simulink model "FinalProjectSimulinkModel_OBSTACLE"  (R2023b)
settings: Solver=VariableStepAuto  StartTime=0.0  StopTime=17  RelTol=1e-3
values from neighbouring files (symbols this model uses):
  dq_d_COM = [0.75; 0; 0; 0; 0; 0]    [FinalProject_init.m]
  dq_d_COM_Jump = [10; 0; 20; 0; -30; 0]    [FinalProject_init.m]
  dq_d_COM_Jump_2 = [12; 0; 21.2; 0; -35.6; 0]    [FinalProject_init.m]
  dtMPC = 0.03    [FinalProject_init.m]
  firstStairDist = 0.26    [FinalProject_init.m]
  flight_gait_2 = [tcrouch2;fFofft2;rFofft2;rlandt2;flandt2; tImpact]    [FinalProject_init.m]
  flight_gait_t = [tcrouch;fFofft;rFofft;rlandt;flandt; tImpact]    [FinalProject_init.m]
  kd_swing = 10    [FinalProject_init.m]
  kp_swing = 300    [FinalProject_init.m]
  kStep = 0.001    [FinalProject_init.m]
  NMPC = 10    [FinalProject_init.m]
  offsets = [0;tSwing;tSwing;0]    [FinalProject_init.m]
  q_d_crouch = [q_hip_roll_f ... (first row only)    [FinalProject_init.m]
  q_d_impact = [q_hip_roll_i_f ... (first row only)    [FinalProject_init.m]
  q_d_stand = [q_hip_roll_i;q_hip_pitch_i;q_knee_i]    [FinalProject_init.m]
  q_hip_roll_i = 0    [FinalProject_init.m]
  Qmpc = diag([100 100 50 1000 1000 500 4 4 4 1 1 1 0])    [FinalProject_init.m]
  rFofft = 0.12+tcrouch    (= 1.12)    [FinalProject_init.m]
  rFofft2 = 0.12+tcrouch2    (= 1.42)    [FinalProject_init.m]
  Rmpc = 0.00001*eye(12)    [FinalProject_init.m]
  task = 6    [FinalProject_init.m]
  tcrouch = 1.0    (= 1)    [FinalProject_init.m]
  tcrouch2 = 1.3    [FinalProject_init.m]
  tCycle = 0.3    [FinalProject_init.m]
  tRamp = 0.5    [FinalProject_init.m]
  tRamp_Jump = 0.05    [FinalProject_init.m]
  tRamp_Jump2 = 0.08    [FinalProject_init.m]
  tSlow = 0.3    [FinalProject_init.m]
  tSwing = tCycle/2    (= 0.15)    [FinalProject_init.m]
  x0_Trunk = [0;0;z_trunk_i-.15; 0;-0.271;0]    [FinalProject_init.m]
undefined symbols (not defined in the file or in its folder): kStepTheta, X, Y, Z
libraries: sm_lib x199, nesl_utility x53
(part 1 of 6)
settings Model: Creator=Scott  LastModifiedBy=Scott

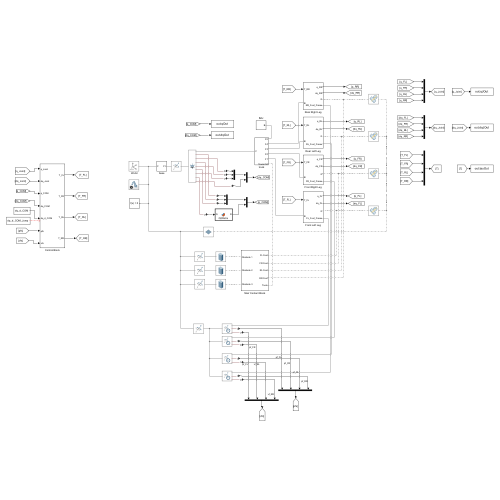
[thumbnail: Simulink's stored preview of the top-level diagram]
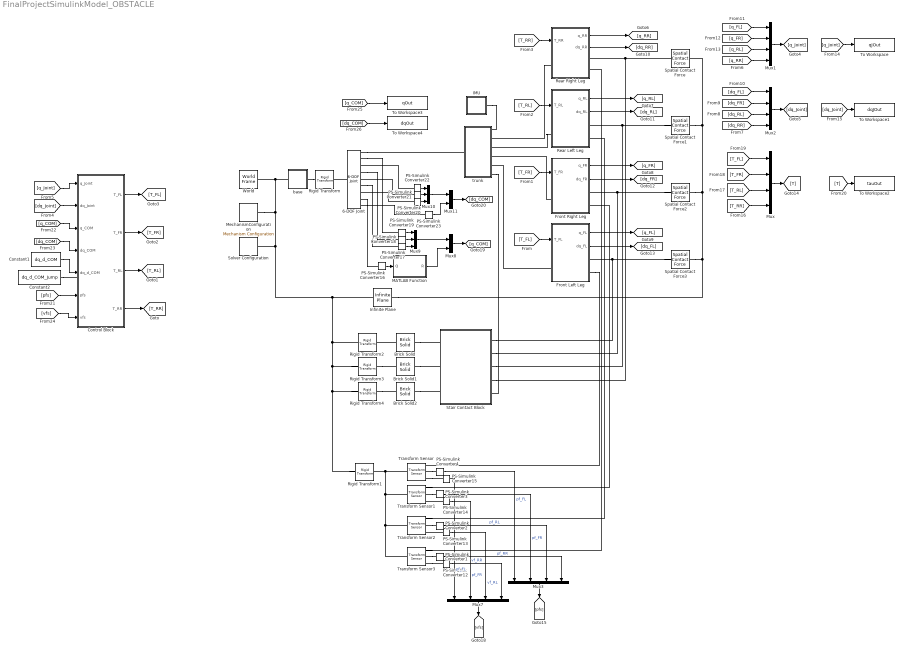
== system FinalProjectSimulinkModel_OBSTACLE ==
  6-DOF Joint : sm_lib/Joints/6-DOF Joint  JointMode=Normal  SenseConstraintForce=off  SenseConstraintForceX=off  SenseConstraintForceY=off  SenseConstraintForceZ=off  SenseConstraintTorque=off  SenseConstraintTorqueX=off  SenseConstraintTorqueY=off  SenseConstraintTorqueZ=off  SenseTotalForce=off  SenseTotalForceX=off  SenseTotalForceY=off  SenseTotalForceZ=off  SenseTotalTorque=off  SenseTotalTorqueX=off  SenseTotalTorqueY=off  SenseTotalTorqueZ=off  CompositeWrenchDir=FollowerOnBase  CompositeWrenchFrame=BaseFrame  PxEquilibriumPosition=0  PxEquilibriumPositionUnits=m  PxSpringStiffness=0  PxSpringStiffnessUnits=N/m  PxDampingCoefficient=0  PxDampingCoefficientUnits=N/(m/s)  PxTorqueActuationMode=NoTorque  PxMotionActuationMode=ComputedMotion  PxSensePosition=on  PxSenseVelocity=on  PxSenseAcceleration=off  PxSenseTorqueForce=off  PxSenseLowerLimitTorqueForce=off  PxSenseUpperLimitTorqueForce=off  PxLowerLimitSpecify=off  PxLowerLimitBound=-1  PxLowerLimitBoundUnits=m  PxLowerLimitStiffness=1e6  PxLowerLimitStiffnessUnits=N/m  PxLowerLimitDamping=1e3  PxLowerLimitDampingUnits=N/(m/s)  PxLowerLimitTransitionRegionWidth=1e-4  PxLowerLimitTransitionRegionWidthUnits=m  PxUpperLimitSpecify=off  PxUpperLimitBound=1  PxUpperLimitBoundUnits=m  PxUpperLimitStiffness=1e6  PxUpperLimitStiffnessUnits=N/m  PxUpperLimitDamping=1e3  PxUpperLimitDampingUnits=N/(m/s)  PxUpperLimitTransitionRegionWidth=1e-4  PxUpperLimitTransitionRegionWidthUnits=m  PxPositionTargetSpecify=off  PxPositionTargetPriority=High  PxPositionTargetValue=0  PxPositionTargetValueUnits=m  PxVelocityTargetSpecify=off  PxVelocityTargetPriority=High  PxVelocityTargetValue=0  PxVelocityTargetValueUnits=m/s  PyEquilibriumPosition=0  PyEquilibriumPositionUnits=m  PySpringStiffness=0  PySpringStiffnessUnits=N/m  PyDampingCoefficient=0  PyDampingCoefficientUnits=N/(m/s)  PyTorqueActuationMode=NoTorque  PyMotionActuationMode=ComputedMotion  PySensePosition=on  PySenseVelocity=on  PySenseAcceleration=off  PySenseTorqueForce=off  PySenseLowerLimitTorqueForce=off  PySenseUpperLimitTorqueForce=off  PyLowerLimitSpecify=off  PyLowerLimitBound=-1  PyLowerLimitBoundUnits=m  PyLowerLimitStiffness=1e6  PyLowerLimitStiffnessUnits=N/m  PyLowerLimitDamping=1e3  PyLowerLimitDampingUnits=N/(m/s)  PyLowerLimitTransitionRegionWidth=1e-4  PyLowerLimitTransitionRegionWidthUnits=m  PyUpperLimitSpecify=off  PyUpperLimitBound=1  PyUpperLimitBoundUnits=m  PyUpperLimitStiffness=1e6  PyUpperLimitStiffnessUnits=N/m  PyUpperLimitDamping=1e3  PyUpperLimitDampingUnits=N/(m/s)  PyUpperLimitTransitionRegionWidth=1e-4  PyUpperLimitTransitionRegionWidthUnits=m  PyPositionTargetSpecify=off  PyPositionTargetPriority=High  PyPositionTargetValue=0  PyPositionTargetValueUnits=m  PyVelocityTargetSpecify=off  PyVelocityTargetPriority=High  PyVelocityTargetValue=0  PyVelocityTargetValueUnits=m/s  PzEquilibriumPosition=0  PzEquilibriumPositionUnits=m  PzSpringStiffness=0  PzSpringStiffnessUnits=N/m  PzDampingCoefficient=0  PzDampingCoefficientUnits=N/(m/s)  PzTorqueActuationMode=NoTorque  PzMotionActuationMode=ComputedMotion  PzSensePosition=on  PzSenseVelocity=on  PzSenseAcceleration=off  PzSenseTorqueForce=off  PzSenseLowerLimitTorqueForce=off  PzSenseUpperLimitTorqueForce=off  PzLowerLimitSpecify=off  PzLowerLimitBound=-1  PzLowerLimitBoundUnits=m  PzLowerLimitStiffness=1e6  PzLowerLimitStiffnessUnits=N/m  PzLowerLimitDamping=1e3  PzLowerLimitDampingUnits=N/(m/s)  PzLowerLimitTransitionRegionWidth=1e-4  PzLowerLimitTransitionRegionWidthUnits=m  PzUpperLimitSpecify=off  PzUpperLimitBound=1  PzUpperLimitBoundUnits=m  PzUpperLimitStiffness=1e6  PzUpperLimitStiffnessUnits=N/m  PzUpperLimitDamping=1e3  PzUpperLimitDampingUnits=N/(m/s)  PzUpperLimitTransitionRegionWidth=1e-4  PzUpperLimitTransitionRegionWidthUnits=m  PzPositionTargetSpecify=on  PzPositionTargetPriority=High  PzPositionTargetValue=z_trunk_i  PzPositionTargetValueUnits=m  PzVelocityTargetSpecify=off  PzVelocityTargetPriority=High  PzVelocityTargetValue=0  PzVelocityTargetValueUnits=m/s  SphEqPosRotationMethod=None  SphEqPosRotationAngleUnits=deg  SphEqPosRotationStandardAxis=+Z  SphEqPosRotationAngle=0.0  SphEqPosRotationArbitraryAxis=[0 0 1]  SphEqPosFollAlignAxisA=+X  SphEqPosBaseAlignAxisA=+Y  SphEqPosFollAlignAxisB=+Y  SphEqPosBaseAlignAxisB=+Z  SphEqPosRotationSequenceAxes=FollowerAxes  SphEqPosRotationSequence=XYX  SphEqPosRotationSequenceAngles=[0 0 0]  SphEqPosRotationSequenceAnglesUnits=deg  SphEqPosRotationMatrix=[1 0 0; 0 1 0; 0 0 1]  SphEqPosQuaternion=[1 0 0 0]  SphSpringStiffness=0  SphSpringStiffnessUnits=N*m/deg  SphDampingCoefficient=0  SphDampingCoefficientUnits=N*m/(deg/s)  SphActuateTorqueX=off  SphActuateTorqueY=off  SphActuateTorqueZ=off  SphActuateTorque=off  SphTorqueActuationMode=NoTorque  SphMotionActuationMode=ComputedMotion  SphActuationFrame=BaseFrame  SphSensePosition=on  SphSenseVelocityX=off  SphSenseVelocityY=off  SphSenseVelocityZ=off  SphSenseVelocity=on  SphSenseAccelerationX=off  SphSenseAccelerationY=off  SphSenseAccelerationZ=off  SphSenseAcceleration=off  SphSenseTorqueX=off  SphSenseTorqueY=off  SphSenseTorqueZ=off  SphSenseTorqueForce=off  SphSenseLowerLimitTorqueMag=off  SphSenseUpperLimitTorqueMag=off  SphSensingFrame=BaseFrame  SphLowerLimitSpecify=off  SphLowerLimitBound=15  SphLowerLimitBoundUnits=deg  SphLowerLimitStiffness=1e4  SphLowerLimitStiffnessUnits=N*m/deg  SphLowerLimitDamping=10  SphLowerLimitDampingUnits=N*m/(deg/s)  SphLowerLimitTransitionRegionWidth=0.1  SphLowerLimitTransitionRegionWidthUnits=deg  SphUpperLimitSpecify=off  SphUpperLimitBound=45  SphUpperLimitBoundUnits=deg  SphUpperLimitStiffness=1e4  SphUpperLimitStiffnessUnits=N*m/deg  SphUpperLimitDamping=10  SphUpperLimitDampingUnits=N*m/(deg/s)  SphUpperLimitTransitionRegionWidth=0.1  SphUpperLimitTransitionRegionWidthUnits=deg  SphPositionTargetRotationMethod=None  SphPositionTargetRotationAngleUnits=deg  SphPositionTargetRotationStandardAxis=+Z  SphPositionTargetRotationAngle=0.0  SphPositionTargetRotationArbitraryAxis=[0 0 1]  SphPositionTargetFollAlignAxisA=+X  SphPositionTargetBaseAlignAxisA=+Y  SphPositionTargetFollAlignAxisB=+Y  SphPositionTargetBaseAlignAxisB=+Z  SphPositionTargetRotationSequenceAxes=FollowerAxes  SphPositionTargetRotationSequence=XYX  SphPositionTargetRotationSequenceAngles=[0 0 0]  SphPositionTargetRotationSequenceAnglesUnits=deg  SphPositionTargetRotationMatrix=[1 0 0; 0 1 0; 0 0 1]  SphPositionTargetQuaternion=[1 0 0 0]  SphPositionTargetSpecify=off  SphPositionTargetPriority=High  SphVelocityTargetValue=[0 0 0]  SphVelocityTargetValueUnits=deg/s  SphVelocityTargetSpecify=off  SphVelocityTargetPriority=High  SphVelocityTargetInFollowerFrame=on
  Brick Solid : sm_lib/Body Elements/Brick Solid  GraphicAmbientColor=[0.15 0.15 0.15 1.0]  BasedOnType=Density  BrickDimensions=[.8 2 .2]  BrickDimensionsUnits=m  CenterOfMass=[0 0 0]  CenterOfMassUnits=m  GraphicDiffuseColor=[0.5 0.5 0.5]  Density=1000  DensityUnits=kg/m^3  DoExposeReferenceFrame=off  GraphicEmissiveColor=[0.0 0.0 0.0 1.0]  ExportEntireGeometry=on  SerializedFrames=<Frames><Frame><Id>Frame1</Id><Value><Name>F1</Name><Origin><Source>GeometricFeature</Source><FeatureName>-z -x curve</FeatureName></Origin><PrimaryAxis><DefinedDirection>+Z</DefinedDirection><Source>ReferenceFrame</Source><SourceDirection>+Z</SourceDirection><FeatureName></FeatureName></PrimaryAxis><SecondaryAxis><DefinedDirection>+X</DefinedDirection><Source>ReferenceFrame</Source><SourceDirection>+X</SourceDirection><FeatureName></FeatureName></SecondaryAxis></Value></Frame></Frames>  MarkerShape=Sphere  MarkerSize=10  GraphicType=FromGeometry  InertiaType=CalculateFromGeometry  Mass=1  MassUnits=kg  MomentsOfInertia=[1 1 1]  MomentsOfInertiaUnits=kg*m^2  GraphicOpacity=1.0  ProductsOfInertia=[0 0 0]  ProductsOfInertiaUnits=kg*m^2  GraphicShininess=75  GraphicSpecularColor=[0.5 0.5 0.5 1.0]  GraphicVisPropType=SimpleVisualProperties
  Brick Solid1 : sm_lib/Body Elements/Brick Solid  GraphicAmbientColor=[0.15 0.15 0.15 1.0]  BasedOnType=Density  BrickDimensions=[3 2 1]  BrickDimensionsUnits=m  CenterOfMass=[0 0 0]  CenterOfMassUnits=m  GraphicDiffuseColor=[0.5 0.5 0.5]  Density=1000  DensityUnits=kg/m^3  DoExposeReferenceFrame=off  GraphicEmissiveColor=[0.0 0.0 0.0 1.0]  ExportEntireGeometry=on  SerializedFrames=<Frames><Frame><Id>Frame1</Id><Value><Name>F1</Name><Origin><Source>GeometricFeature</Source><FeatureName>-z -x curve</FeatureName></Origin><PrimaryAxis><DefinedDirection>+Z</DefinedDirection><Source>ReferenceFrame</Source><SourceDirection>+Z</SourceDirection><FeatureName></FeatureName></PrimaryAxis><SecondaryAxis><DefinedDirection>+X</DefinedDirection><Source>ReferenceFrame</Source><SourceDirection>+X</SourceDirection><FeatureName></FeatureName></SecondaryAxis></Value></Frame></Frames>  MarkerShape=Sphere  MarkerSize=10  GraphicType=FromGeometry  InertiaType=CalculateFromGeometry  Mass=1  MassUnits=kg  MomentsOfInertia=[1 1 1]  MomentsOfInertiaUnits=kg*m^2  GraphicOpacity=1.0  ProductsOfInertia=[0 0 0]  ProductsOfInertiaUnits=kg*m^2  GraphicShininess=75  GraphicSpecularColor=[0.5 0.5 0.5 1.0]  GraphicVisPropType=SimpleVisualProperties
  Brick Solid2 : sm_lib/Body Elements/Brick Solid  GraphicAmbientColor=[0.15 0.15 0.15 1.0]  BasedOnType=Density  BrickDimensions=[.2 2 .5]  BrickDimensionsUnits=m  CenterOfMass=[0 0 0]  CenterOfMassUnits=m  GraphicDiffuseColor=[0.5 0.5 0.5]  Density=1000  DensityUnits=kg/m^3  DoExposeReferenceFrame=off  GraphicEmissiveColor=[0.0 0.0 0.0 1.0]  ExportEntireGeometry=on  SerializedFrames=<Frames><Frame><Id>Frame1</Id><Value><Name>F1</Name><Origin><Source>GeometricFeature</Source><FeatureName>-z -x curve</FeatureName></Origin><PrimaryAxis><DefinedDirection>+Z</DefinedDirection><Source>ReferenceFrame</Source><SourceDirection>+Z</SourceDirection><FeatureName></FeatureName></PrimaryAxis><SecondaryAxis><DefinedDirection>+X</DefinedDirection><Source>ReferenceFrame</Source><SourceDirection>+X</SourceDirection><FeatureName></FeatureName></SecondaryAxis></Value></Frame></Frames>  MarkerShape=Sphere  MarkerSize=10  GraphicType=FromGeometry  InertiaType=CalculateFromGeometry  Mass=1  MassUnits=kg  MomentsOfInertia=[1 1 1]  MomentsOfInertiaUnits=kg*m^2  GraphicOpacity=1.0  ProductsOfInertia=[0 0 0]  ProductsOfInertiaUnits=kg*m^2  GraphicShininess=75  GraphicSpecularColor=[0.5 0.5 0.5 1.0]  GraphicVisPropType=SimpleVisualProperties
  Constant1 : Constant  Value=dq_d_COM
  Constant2 : Constant  Value=dq_d_COM_Jump
  Control Block : Subsystem
  Front Left Leg : Subsystem
  Front Right Leg : Subsystem
  IMU : Subsystem
  Infinite Plane : sm_lib/Curves and Surfaces/Infinite Plane  GraphicType=Rectangle  GraphicPlaneWidth=1  GraphicPlaneWidthUnits=m  GraphicPlaneHeight=1  GraphicPlaneHeightUnits=m  GraphicVisPropType=SimpleVisualProperties  GraphicDiffuseColor=[0.5 0.5 0.5]  GraphicOpacity=0.25  GraphicSpecularColor=[0.5 0.5 0.5 1.0]  GraphicAmbientColor=[0.15 0.15 0.15 1.0]  GraphicEmissiveColor=[0.0 0.0 0.0 1.0]  GraphicShininess=75
  MATLAB Function : MATLAB Function  TreatAsAtomicUnit=on
  MechanismConfiguration : sm_lib/Utilities/Mechanism Configuration  UniformGravity=Constant  GravityVector=[0 0 -9.80665]  GravityVectorUnits=m/s^2  LinearizationDelta=0.001  JointModeTransitionNonlinearIterations=2
  Mux{,1..3,7} (5 alike) : Mux
  Mux10 : Mux  Inputs=3
  Mux11 : Mux  Inputs=2
  Mux8 : Mux  Inputs=2
  Mux9 : Mux  Inputs=3
  PS-Simulink Converter{1..4,12..23} (16 alike) : nesl_utility/PS-Simulink Converter  PhysicalDomain=network_engine_domain  SubClassName=ps_output  LeftPortType=input  RightPortType=output  PseudoPeriodic=off  Frequencies=[]  VectorFormat=inherit  Unit=inherit  AffineConversion=off
  Rear Left Leg : Subsystem
  Rear Right Leg : Subsystem
  Rigid Transform : sm_lib/Frames and Transforms/Rigid Transform  TranslationMethod=StandardAxis  TranslationStandardOffset=0  TranslationStandardOffsetUnits=m  TranslationStandardAxis=+Z  TranslationCartesianOffset=[0 0 0]  TranslationCartesianOffsetUnits=m  TranslationROffset=0  TranslationROffsetUnits=m  TranslationZOffset=0  TranslationZOffsetUnits=m  TranslationThetaOffset=0  TranslationThetaOffsetUnits=deg  RotationMethod=None  RotationAngleUnits=deg  RotationStandardAxis=+Z  RotationAngle=0.0  RotationArbitraryAxis=[0 0 1]  FollAlignAxisA=+X  BaseAlignAxisA=+Y  FollAlignAxisB=+Y  BaseAlignAxisB=+Z  RotationSequenceAxes=FollowerAxes  RotationSequence=XYX  RotationSequenceAngles=[0 0 0]  RotationSequenceAnglesUnits=deg  RotationMatrix=[1 0 0; 0 1 0; 0 0 1]  Quaternion=[1 0 0 0]
  Rigid Transform1 : sm_lib/Frames and Transforms/Rigid Transform  TranslationMethod=StandardAxis  TranslationStandardOffset=0.02  TranslationStandardOffsetUnits=m  TranslationStandardAxis=+Z  TranslationCartesianOffset=[0 0 0]  TranslationCartesianOffsetUnits=m  TranslationROffset=0  TranslationROffsetUnits=m  TranslationZOffset=0  TranslationZOffsetUnits=m  TranslationThetaOffset=0  TranslationThetaOffsetUnits=deg  RotationMethod=None  RotationAngleUnits=deg  RotationStandardAxis=+Z  RotationAngle=0.0  RotationArbitraryAxis=[0 0 1]  FollAlignAxisA=+X  BaseAlignAxisA=+Y  FollAlignAxisB=+Y  BaseAlignAxisB=+Z  RotationSequenceAxes=FollowerAxes  RotationSequence=XYX  RotationSequenceAngles=[0 0 0]  RotationSequenceAnglesUnits=deg  RotationMatrix=[1 0 0; 0 1 0; 0 0 1]  Quaternion=[1 0 0 0]
  Rigid Transform2 : sm_lib/Frames and Transforms/Rigid Transform  TranslationMethod=Cartesian  TranslationStandardOffset=0.02  TranslationStandardOffsetUnits=m  TranslationStandardAxis=+Z  TranslationCartesianOffset=[1 0 .0]  TranslationCartesianOffsetUnits=m  TranslationROffset=0  TranslationROffsetUnits=m  TranslationZOffset=0  TranslationZOffsetUnits=m  TranslationThetaOffset=0  TranslationThetaOffsetUnits=deg  RotationMethod=None  RotationAngleUnits=deg  RotationStandardAxis=+Z  RotationAngle=0.0  RotationArbitraryAxis=[0 0 1]  FollAlignAxisA=+X  BaseAlignAxisA=+Y  FollAlignAxisB=+Y  BaseAlignAxisB=+Z  RotationSequenceAxes=FollowerAxes  RotationSequence=XYX  RotationSequenceAngles=[0 0 0]  RotationSequenceAnglesUnits=deg  RotationMatrix=[1 0 0; 0 1 0; 0 0 1]  Quaternion=[1 0 0 0]
  Rigid Transform3 : sm_lib/Frames and Transforms/Rigid Transform  TranslationMethod=Cartesian  TranslationStandardOffset=0.02  TranslationStandardOffsetUnits=m  TranslationStandardAxis=+Z  TranslationCartesianOffset=[2.8 0 0.35]  TranslationCartesianOffsetUnits=m  TranslationROffset=0  TranslationROffsetUnits=m  TranslationZOffset=0  TranslationZOffsetUnits=m  TranslationThetaOffset=0  TranslationThetaOffsetUnits=deg  RotationMethod=None  RotationAngleUnits=deg  RotationStandardAxis=+Z  RotationAngle=0.0  RotationArbitraryAxis=[0 0 1]  FollAlignAxisA=+X  BaseAlignAxisA=+Y  FollAlignAxisB=+Y  BaseAlignAxisB=+Z  RotationSequenceAxes=FollowerAxes  RotationSequence=XYX  RotationSequenceAngles=[0 0 0]  RotationSequenceAnglesUnits=deg  RotationMatrix=[1 0 0; 0 1 0; 0 0 1]  Quaternion=[1 0 0 0]
  Rigid Transform4 : sm_lib/Frames and Transforms/Rigid Transform  TranslationMethod=Cartesian  TranslationStandardOffset=0.02  TranslationStandardOffsetUnits=m  TranslationStandardAxis=+Z  TranslationCartesianOffset=[6.8 0 0]  TranslationCartesianOffsetUnits=m  TranslationROffset=0  TranslationROffsetUnits=m  TranslationZOffset=0  TranslationZOffsetUnits=m  TranslationThetaOffset=0  TranslationThetaOffsetUnits=deg  RotationMethod=None  RotationAngleUnits=deg  RotationStandardAxis=+Z  RotationAngle=0.0  RotationArbitraryAxis=[0 0 1]  FollAlignAxisA=+X  BaseAlignAxisA=+Y  FollAlignAxisB=+Y  BaseAlignAxisB=+Z  RotationSequenceAxes=FollowerAxes  RotationSequence=XYX  RotationSequenceAngles=[0 0 0]  RotationSequenceAnglesUnits=deg  RotationMatrix=[1 0 0; 0 1 0; 0 0 1]  Quaternion=[1 0 0 0]
  Solver Configuration : nesl_utility/Solver Configuration  PhysicalDomain=network_engine_domain  SubClassName=solver  LeftPortType=input  RightPortType=generic  Tones=[]  Harmonics=[]  SimulateNoise=off  Profile=off  UseLocalSampling=off  EnableSwitchedLinearOptims=on  FrequencyDomain=off  UseCCode=off  RelTol=0.001  AbsTol=0.001  MinStep=1e-09  ToWorkspace=off  RevertToSquareIcSolve=off  NumHomotopyIterations=100  PhasorMode=off  PhasorModeNumHarmonics=1  ConsistencySolver=NEWTON_XTOL_AFTER_FTOL  IndexReductionMethod=DerivativeReplacement  DoDC=off  ResidualTolerance=1e-09  ConsistencyTolSource=GLOBAL  ConsistencyAbsTol=0.001  ConsistencyRelTol=0.001  ConsistencyTolFactor=0.001  UseLocalSolver=off  LocalSolverChoice=NE_BACKWARD_EULER_ADVANCER  ResolveIndetEquations=on  FunctionEvalNumThread=1  LocalSolverSampleTime=0.001  DoFixedCost=off  MaxNonlinIter=3  MaxModeIter=2  ComputeImpulses=off  ImpulseIterations=2  LinearAlgebra=auto  LinearAlgebraNumThread=0  EquationFormulation=NE_TIME_EF  DelaysMemoryBudget=1024  AutomaticFiltering=on  FilteringTimeConstant=0.001  PartitionStorageMethod=AS_NEEDED  PartitionMemoryBudget=1024  PartitionMethod=ROBUST  MultibodyUseLocalSolver=off  MultibodyLocalSolverChoice=ODE1  MultibodyLocalSolverSampleTime=0.001
  Spatial Contact Force{,1..3} (4 alike) : sm_lib/Forces and Torques/Spatial Contact Force  SenseContactBaseRotation=off  SenseContactBaseTranslation=off  CoefficientOfDynamicFriction=0.5  CoefficientOfStaticFriction=0.5  NormalDamping=1e3  NormalDampingUnits=N/(m/s)  SenseContactSignal=off  NormalStiffness=1e6  NormalStiffnessUnits=N/m  FrictionalCriticalVelocity=1e-3  FrictionalCriticalVelocityUnits=m/s  ZeroCrossDetectContactStartAndEnd=off  SenseContactFollowerRotation=off  SenseContactFollowerTranslation=off  FrictionType=SmoothStickSlip  SenseFrictionalForceMagnitude=off  SenseNormalForceMagnitude=off  NormalForceType=SmoothSpringDamper  SenseNormalVelocity=off  SensePenetrationDepth=off  SenseSeparationDistance=off  SenseTangentialVelocity=off  NormalTransitionRegionWidth=1e-4  NormalTransitionRegionWidthUnits=m
  Stair Contact Block : Subsystem
  To Workspace : ToWorkspace  VariableName=qJOut  SampleTime=-1
  To Workspace1 : ToWorkspace  VariableName=dqJOut  SampleTime=-1
  To Workspace2 : ToWorkspace  VariableName=tauOut  SampleTime=-1
  To Workspace3 : ToWorkspace  VariableName=qOut  SampleTime=-1
  To Workspace4 : ToWorkspace  VariableName=dqOut  SampleTime=-1
  Transform Sensor{,1..3} (4 alike) : sm_lib/Frames and Transforms/Transform Sensor  MeasurementFrame=World  RotationSequence=XYX  SenseAngle=off  SenseAxis=off  SenseQ=off  SenseR=off  SenseRotationSequence=off  SenseOmegaX=off  SenseOmegaY=off  SenseOmegaZ=off  SenseOmega=off  SenseQDot=off  SenseRDot=off  SenseRotationSequenceDot=off  SenseAlphaX=off  SenseAlphaY=off  SenseAlphaZ=off  SenseAlpha=off  SenseQDDot=off  SenseRDDot=off  SenseX=off  SenseY=off  SenseZ=off  SenseXYZ=on  SenseRad=off  SenseAzim=off  SenseDist=off  SenseInc=off  SenseXDot=off  SenseYDot=off  SenseZDot=off  SenseXYZDot=on  SenseRadDot=off  SenseAzimDot=off  SenseDistDot=off  SenseIncDot=off  SenseXDDot=off  SenseYDDot=off  SenseZDDot=off  SenseXYZDDot=off  SenseRadDDot=off  SenseAzimDDot=off  SenseDistDDot=off  SenseIncDDot=off
  World : sm_lib/Frames and Transforms/World Frame
  base : Subsystem
  trunk : Subsystem
  wires:
  [T_FL] -> Front Left Leg/1(T_FL)
  [T_FR] -> Front Right Leg/1(T_FR)
  [T_RL] -> Rear Left Leg/1(T_RL)
  [T_RR] -> Rear Right Leg/1(T_RR)
  [q_Joint] -> Control Block/1(q_Joint)
  Rear Right Leg/1(q_RR) -> [q_RR]
  Rear Right Leg/2(dq_RR) -> [dq_RR]
  Rear Left Leg/1(q_RL) -> [q_RL]
  Rear Left Leg/2(dq_RL) -> [dq_RL]
  Front Right Leg/2(dq_FR) -> [dq_FR]
  Front Right Leg/1(q_FR) -> [q_FR]
  Front Left Leg/1(q_FL) -> [q_FL]
  Front Left Leg/2(dq_FL) -> [dq_FL]
  Mux1/1 -> [q_Joint]
  Mux2/1 -> [dq_Joint]
  [q_Joint] -> To Workspace/1
  [dq_Joint] -> To Workspace1/1
  Mux/1 -> [T]
  [T] -> To Workspace2/1
  PS-Simulink Converter1/1 -> Mux3/4  "pf_RR"
  PS-Simulink Converter2/1 -> Mux3/3  "pf_RL"
  PS-Simulink Converter3/1 -> Mux3/2  "pf_FR"
  PS-Simulink Converter4/1 -> Mux3/1  "pf_FL"
  Mux3/1 -> [pfs]
  Control Block/1(T_FL) -> [T_FL]
  [dq_Joint] -> Control Block/2(dq_Joint)
  Constant1/1 -> Control Block/5(dq_d_COM)
  Control Block/4(T_RR) -> [T_RR]
  Control Block/3(T_RL) -> [T_RL]
  Control Block/2(T_FR) -> [T_FR]
  [pfs] -> Control Block/6(pfs)
  [q_COM] -> Control Block/3(q_COM)
  [dq_COM] -> Control Block/4(dq_COM)
  [dq_RL] -> Mux2/3
  [dq_RR] -> Mux2/4
  [dq_FR] -> Mux2/2
  [dq_FL] -> Mux2/1
  [q_RL] -> Mux1/3
  [q_RR] -> Mux1/4
  [q_FR] -> Mux1/2
  [q_FL] -> Mux1/1
  [T_FL] -> Mux/1
  [T_FR] -> Mux/2
  [T_RL] -> Mux/3
  [T_RR] -> Mux/4
  Mux7/1 -> [vfs]
  PS-Simulink Converter14/1 -> Mux7/2  "pf_FR"
  PS-Simulink Converter13/1 -> Mux7/3  "vf_RL"
  PS-Simulink Converter15/1 -> Mux7/1  "pf_FL"
  PS-Simulink Converter12/1 -> Mux7/4  "vf_RR"
  [vfs] -> Control Block/7(vfs)
  [dq_COM] -> To Workspace4/1
  [q_COM] -> To Workspace3/1
  PS-Simulink Converter16/1 -> MATLAB Function/1(Q)
  PS-Simulink Converter19/1 -> Mux9/1
  PS-Simulink Converter18/1 -> Mux9/2
  PS-Simulink Converter17/1 -> Mux9/3
  PS-Simulink Converter20/1 -> Mux10/3
  PS-Simulink Converter21/1 -> Mux10/2
  PS-Simulink Converter22/1 -> Mux10/1
  MATLAB Function/1(R) -> Mux8/2
  Mux8/1 -> [q_COM]
  Mux11/1 -> [dq_COM]
  Mux10/1 -> Mux11/1
  Mux9/1 -> Mux8/1
  PS-Simulink Converter23/1 -> Mux11/2
  Constant2/1 -> ?
  connections:
  6-DOF Joint/LConn1 -- Rigid Transform/RConn1
  6-DOF Joint/RConn1 -- trunk/LConn1
  MechanismConfiguration/RConn1 -- Rigid Transform1/LConn1 -- Rigid Transform4/LConn1 -- Rigid Transform3/LConn1 -- Rigid Transform2/LConn1 -- Infinite Plane/LConn1 -- Solver Configuration/RConn1 -- World/RConn1 -- base/LConn1
  IMU/LConn1 -- trunk/RConn1
  Rear Right Leg/LConn1 -- trunk/RConn2
  Rear Left Leg/LConn1 -- trunk/RConn3
  Front Right Leg/LConn1 -- trunk/RConn4
  Front Left Leg/LConn1 -- trunk/RConn5
  Spatial Contact Force1/LConn1 -- Rear Left Leg/RConn1 -- Stair Contact Block/RConn3
  Spatial Contact Force/LConn1 -- Rear Right Leg/RConn1 -- Stair Contact Block/RConn4
  Spatial Contact Force2/LConn1 -- Front Right Leg/RConn1 -- Stair Contact Block/RConn2
  Spatial Contact Force3/LConn1 -- Front Left Leg/RConn1 -- Stair Contact Block/RConn1
  Infinite Plane/RConn1 -- Spatial Contact Force3/RConn1 -- Spatial Contact Force2/RConn1 -- Spatial Contact Force1/RConn1 -- Spatial Contact Force/RConn1
  base/RConn1 -- Rigid Transform/LConn1
  Transform Sensor1/RConn1 -- Front Right Leg/RConn2
  Transform Sensor2/RConn1 -- Rear Left Leg/RConn2
  Transform Sensor/RConn2 -- PS-Simulink Converter4/LConn1
  Transform Sensor1/RConn2 -- PS-Simulink Converter3/LConn1
  Transform Sensor2/RConn2 -- PS-Simulink Converter2/LConn1
  Transform Sensor3/RConn2 -- PS-Simulink Converter1/LConn1
  Front Left Leg/RConn2 -- Transform Sensor/RConn1
  Transform Sensor3/RConn1 -- Rear Right Leg/RConn2
  Transform Sensor3/RConn3 -- PS-Simulink Converter12/LConn1
  PS-Simulink Converter13/LConn1 -- Transform Sensor2/RConn3
  PS-Simulink Converter14/LConn1 -- Transform Sensor1/RConn3
  Transform Sensor/RConn3 -- PS-Simulink Converter15/LConn1
  Transform Sensor/LConn1 -- Transform Sensor2/LConn1 -- Transform Sensor3/LConn1 -- Transform Sensor1/LConn1 -- Rigid Transform1/RConn1
  6-DOF Joint/RConn8 -- PS-Simulink Converter16/LConn1
  6-DOF Joint/RConn2 -- PS-Simulink Converter19/LConn1
  6-DOF Joint/RConn4 -- PS-Simulink Converter18/LConn1
  6-DOF Joint/RConn6 -- PS-Simulink Converter17/LConn1
  PS-Simulink Converter20/LConn1 -- 6-DOF Joint/RConn7
  PS-Simulink Converter22/LConn1 -- 6-DOF Joint/RConn3
  PS-Simulink Converter21/LConn1 -- 6-DOF Joint/RConn5
  6-DOF Joint/RConn9 -- PS-Simulink Converter23/LConn1
  Rigid Transform3/RConn1 -- Brick Solid1/LConn1
  Rigid Transform4/RConn1 -- Brick Solid2/LConn1
  Brick Solid/LConn1 -- Rigid Transform2/RConn1
  Brick Solid/RConn1 -- Stair Contact Block/LConn1
  Brick Solid1/RConn1 -- Stair Contact Block/LConn2
  Brick Solid2/RConn1 -- Stair Contact Block/LConn3
  trunk/RConn6 -- Stair Contact Block/RConn5

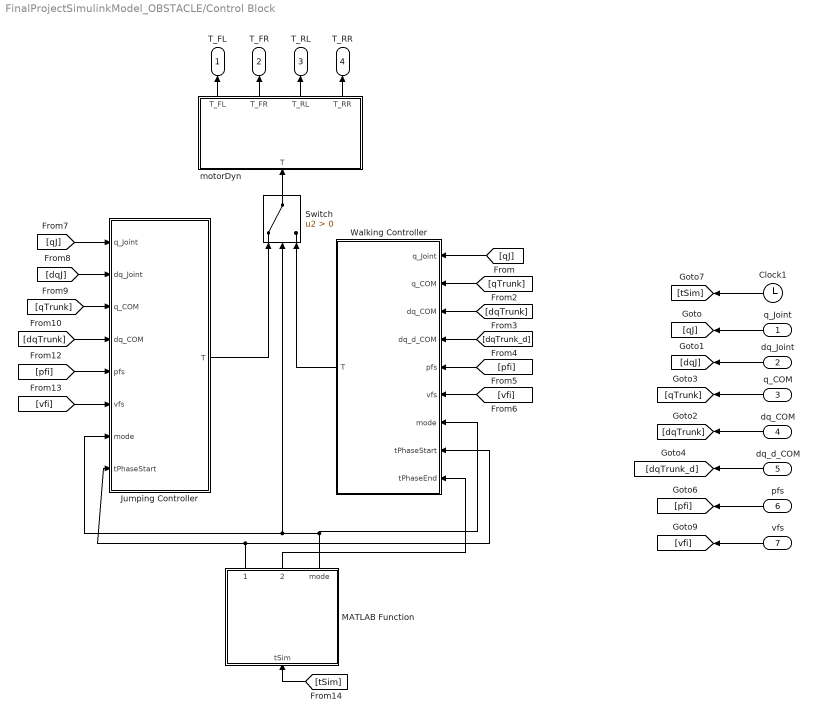
== system FinalProjectSimulinkModel_OBSTACLE/Control Block ==
  q_Joint : Inport
  dq_Joint : Inport  Port=2
  q_COM : Inport  Port=3
  dq_COM : Inport  Port=4
  dq_d_COM : Inport  Port=5
  pfs : Inport  Port=6
  vfs : Inport  Port=7
  Clock1 : Clock
  Jumping Controller : Subsystem
  MATLAB Function : MATLAB Function  TreatAsAtomicUnit=on
  Switch : Switch  Criteria=u2 > Threshold  SaturateOnIntegerOverflow=off  InputSameDT=off
  Walking Controller : Subsystem
  motorDyn : MATLAB Function  TreatAsAtomicUnit=on
  T_FL : Outport
  T_FR : Outport  Port=2
  T_RL : Outport  Port=3
  T_RR : Outport  Port=4
  wires:
  motorDyn/1(T_FL) -> T_FL/1
  motorDyn/3(T_RL) -> T_RL/1
  motorDyn/2(T_FR) -> T_FR/1
  motorDyn/4(T_RR) -> T_RR/1
  q_Joint/1 -> [qJ]
  dq_Joint/1 -> [dqJ]
  q_COM/1 -> [qTrunk]
  dq_COM/1 -> [dqTrunk]
  dq_d_COM/1 -> [dqTrunk_d]
  pfs/1 -> [pfi]
  Clock1/1 -> [tSim]
  vfs/1 -> [vfi]
  [qJ] -> Walking Controller/1(q_Joint)
  [vfi] -> Walking Controller/6(vfs)
  [pfi] -> Walking Controller/5(pfs)
  [dqTrunk_d] -> Walking Controller/4(dq_d_COM)
  [dqTrunk] -> Walking Controller/3(dq_COM)
  [qTrunk] -> Walking Controller/2(q_COM)
  [vfi] -> Jumping Controller/6(vfs)
  [pfi] -> Jumping Controller/5(pfs)
  [dqTrunk] -> Jumping Controller/4(dq_COM)
  [qTrunk] -> Jumping Controller/3(q_COM)
  [dqJ] -> Jumping Controller/2(dq_Joint)
  [qJ] -> Jumping Controller/1(q_Joint)
  MATLAB Function/3(mode) -> Jumping Controller/7(mode), Switch/2, Walking Controller/7(mode)
  Switch/1 -> motorDyn/1(T)
  [tSim] -> MATLAB Function/1(tSim)
  MATLAB Function/1(tPhaseStart) -> Jumping Controller/8(tPhaseStart), Walking Controller/8(tPhaseStart)
  Jumping Controller/1(T) -> Switch/1
  Walking Controller/1(T) -> Switch/3
  MATLAB Function/2(tPhaseEnd) -> Walking Controller/9(tPhaseEnd)

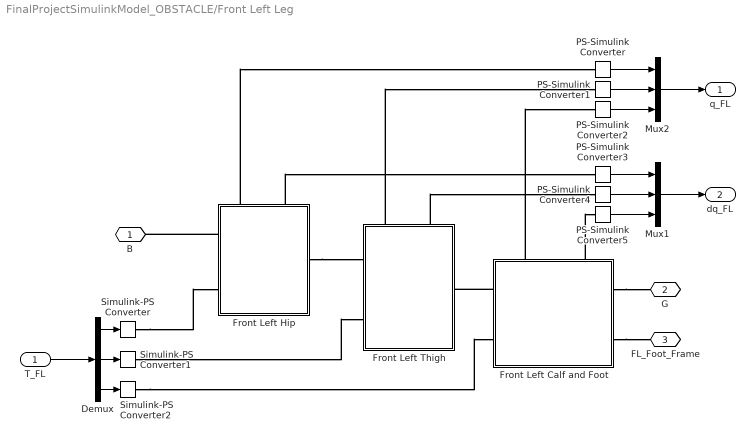
== system FinalProjectSimulinkModel_OBSTACLE/Front Left Leg ==
  T_FL : Inport
  Demux : Demux  Outputs=3
  Front Left Calf and Foot : Subsystem
      settings: PortSchema="{\"entries\":[{\"content\":{\"sides\":[{\"content\":{\"connectorIds\":[\"LConn1\",\"LConn2\"]},\"type\":\"ConnectorPlacement.EquallySpacedRectSide\",\"uuid\":\"13a04993-3104-4ff0-9790-56bc88fd7271\"},{\"content\":{\"connectorIds\":[\"RConn1\",\"RConn2\"],\"side\":\"RIGHT\"},\"type\":\"ConnectorPlacement.EquallySpacedRectSide\",\"uuid\":\"d3121ca2-0bb7-489c-ba63-99aa3bb6178a\"},{\"content\":{\"connectorIds\":[\"LConn3\",\"LConn4\"],\"side\":\"TOP\"},\"type\":\"ConnectorPlacement.EquallySpacedRectSide\",\"uuid\":\"ab9f1076-a7cc-4a5f-a71c-70d0f5e5f642\"}]},\"type\":\"ConnectorPlacement.EquallySpacedConnector\",\"uuid\":\"928155dc-f631-4629-bc1b-5a14a53f9ea7\"}],\"packageUris\":[\"http://schema.mathworks.com/mf0/Connector/R2020b\"],\"version\":\"1.0\"}"
  Front Left Thigh : Subsystem
      settings: PortSchema="{\"entries\":[{\"content\":{\"sides\":[{\"content\":{\"connectorIds\":[\"LConn1\",\"LConn2\"]},\"type\":\"ConnectorPlacement.EquallySpacedRectSide\",\"uuid\":\"13a04993-3104-4ff0-9790-56bc88fd7271\"},{\"content\":{\"connectorIds\":[\"RConn1\"],\"side\":\"RIGHT\"},\"type\":\"ConnectorPlacement.EquallySpacedRectSide\",\"uuid\":\"d3121ca2-0bb7-489c-ba63-99aa3bb6178a\"},{\"content\":{\"connectorIds\":[\"LConn3\",\"LConn4\"],\"side\":\"TOP\"},\"type\":\"ConnectorPlacement.EquallySpacedRectSide\",\"uuid\":\"ab9f1076-a7cc-4a5f-a71c-70d0f5e5f642\"}]},\"type\":\"ConnectorPlacement.EquallySpacedConnector\",\"uuid\":\"928155dc-f631-4629-bc1b-5a14a53f9ea7\"}],\"packageUris\":[\"http://schema.mathworks.com/mf0/Connector/R2020b\"],\"version\":\"1.0\"}"
  Front Left Hip : Subsystem
      settings: PortSchema="{\"entries\":[{\"content\":{\"sides\":[{\"content\":{\"connectorIds\":[\"LConn1\",\"LConn2\"]},\"type\":\"ConnectorPlacement.EquallySpacedRectSide\",\"uuid\":\"13a04993-3104-4ff0-9790-56bc88fd7271\"},{\"content\":{\"connectorIds\":[\"RConn1\"],\"side\":\"RIGHT\"},\"type\":\"ConnectorPlacement.EquallySpacedRectSide\",\"uuid\":\"d3121ca2-0bb7-489c-ba63-99aa3bb6178a\"},{\"content\":{\"connectorIds\":[\"LConn3\",\"LConn4\"],\"side\":\"TOP\"},\"type\":\"ConnectorPlacement.EquallySpacedRectSide\",\"uuid\":\"ab9f1076-a7cc-4a5f-a71c-70d0f5e5f642\"}]},\"type\":\"ConnectorPlacement.EquallySpacedConnector\",\"uuid\":\"928155dc-f631-4629-bc1b-5a14a53f9ea7\"}],\"packageUris\":[\"http://schema.mathworks.com/mf0/Connector/R2020b\"],\"version\":\"1.0\"}"
  Mux1 : Mux  Inputs=3
  Mux2 : Mux  Inputs=3
  PS-Simulink Converter{,1..5} (6 alike) : nesl_utility/PS-Simulink Converter  PhysicalDomain=network_engine_domain  SubClassName=ps_output  LeftPortType=input  RightPortType=output  PseudoPeriodic=off  Frequencies=[]  VectorFormat=inherit  Unit=inherit  AffineConversion=off
  Simulink-PS Converter : nesl_utility/Simulink-PS Converter  PhysicalDomain=network_engine_domain  SubClassName=ps_input  LeftPortType=input  RightPortType=output  PseudoPeriodic=off  Frequencies=[]  NoiseDistribution=none  NoiseParameters=[]  Unit=1  AffineConversion=off  FilteringAndDerivatives=provide  SimscapeFilterOrder=1  InputFilterTimeConstant=0.001  UdotUserProvided=0
  Simulink-PS Converter1 : nesl_utility/Simulink-PS Converter  PhysicalDomain=network_engine_domain  SubClassName=ps_input  LeftPortType=input  RightPortType=output  PseudoPeriodic=off  Frequencies=[]  NoiseDistribution=none  NoiseParameters=[]  Unit=1  AffineConversion=off  FilteringAndDerivatives=provide  SimscapeFilterOrder=1  InputFilterTimeConstant=0.001  UdotUserProvided=0
  Simulink-PS Converter2 : nesl_utility/Simulink-PS Converter  PhysicalDomain=network_engine_domain  SubClassName=ps_input  LeftPortType=input  RightPortType=output  PseudoPeriodic=off  Frequencies=[]  NoiseDistribution=none  NoiseParameters=[]  Unit=1  AffineConversion=off  FilteringAndDerivatives=provide  SimscapeFilterOrder=1  InputFilterTimeConstant=0.001  UdotUserProvided=0
  B : PMIOPort  Side=Left
  G : PMIOPort  Port=2  Side=Right
  FL_Foot_Frame : PMIOPort  Port=3  Side=Right
  q_FL : Outport
  dq_FL : Outport  Port=2
  wires:
  T_FL/1 -> Demux/1
  Demux/1 -> Simulink-PS Converter/1
  Demux/3 -> Simulink-PS Converter2/1
  Demux/2 -> Simulink-PS Converter1/1
  PS-Simulink Converter5/1 -> Mux1/3
  PS-Simulink Converter3/1 -> Mux1/1
  PS-Simulink Converter1/1 -> Mux2/2
  PS-Simulink Converter4/1 -> Mux1/2
  PS-Simulink Converter2/1 -> Mux2/3
  PS-Simulink Converter/1 -> Mux2/1
  Mux1/1 -> dq_FL/1
  Mux2/1 -> q_FL/1
  connections:
  Front Left Hip/LConn1 -- B/RConn1
  Front Left Hip/RConn1 -- Front Left Thigh/LConn1
  Front Left Calf and Foot/RConn1 -- G/RConn1
  Front Left Calf and Foot/LConn1 -- Front Left Thigh/RConn1
  Simulink-PS Converter/RConn1 -- Front Left Hip/LConn2
  Simulink-PS Converter1/RConn1 -- Front Left Thigh/LConn2
  Simulink-PS Converter2/RConn1 -- Front Left Calf and Foot/LConn2
  Front Left Hip/LConn3 -- PS-Simulink Converter/LConn1
  Front Left Thigh/LConn3 -- PS-Simulink Converter1/LConn1
  Front Left Calf and Foot/LConn3 -- PS-Simulink Converter2/LConn1
  Front Left Calf and Foot/LConn4 -- PS-Simulink Converter5/LConn1
  Front Left Thigh/LConn4 -- PS-Simulink Converter4/LConn1
  Front Left Hip/LConn4 -- PS-Simulink Converter3/LConn1
  Front Left Calf and Foot/RConn2 -- FL_Foot_Frame/RConn1

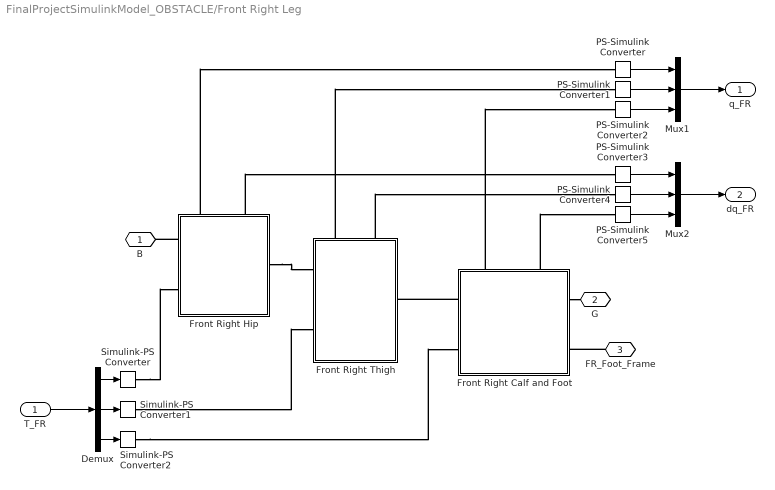
== system FinalProjectSimulinkModel_OBSTACLE/Front Right Leg ==
  T_FR : Inport
  Demux : Demux  Outputs=3
  Front Right Calf and Foot : Subsystem
      settings: PortSchema="{\"entries\":[{\"content\":{\"sides\":[{\"content\":{\"connectorIds\":[\"LConn1\",\"LConn2\"]},\"type\":\"ConnectorPlacement.EquallySpacedRectSide\",\"uuid\":\"13a04993-3104-4ff0-9790-56bc88fd7271\"},{\"content\":{\"connectorIds\":[\"RConn1\",\"RConn2\"],\"side\":\"RIGHT\"},\"type\":\"ConnectorPlacement.EquallySpacedRectSide\",\"uuid\":\"d3121ca2-0bb7-489c-ba63-99aa3bb6178a\"},{\"content\":{\"connectorIds\":[\"LConn3\",\"LConn4\"],\"side\":\"TOP\"},\"type\":\"ConnectorPlacement.EquallySpacedRectSide\",\"uuid\":\"ab9f1076-a7cc-4a5f-a71c-70d0f5e5f642\"}]},\"type\":\"ConnectorPlacement.EquallySpacedConnector\",\"uuid\":\"928155dc-f631-4629-bc1b-5a14a53f9ea7\"}],\"packageUris\":[\"http://schema.mathworks.com/mf0/Connector/R2020b\"],\"version\":\"1.0\"}"
  Front Right Thigh : Subsystem
      settings: PortSchema="{\"entries\":[{\"content\":{\"sides\":[{\"content\":{\"connectorIds\":[\"LConn1\",\"LConn2\"]},\"type\":\"ConnectorPlacement.EquallySpacedRectSide\",\"uuid\":\"13a04993-3104-4ff0-9790-56bc88fd7271\"},{\"content\":{\"connectorIds\":[\"RConn1\"],\"side\":\"RIGHT\"},\"type\":\"ConnectorPlacement.EquallySpacedRectSide\",\"uuid\":\"d3121ca2-0bb7-489c-ba63-99aa3bb6178a\"},{\"content\":{\"connectorIds\":[\"LConn3\",\"LConn4\"],\"side\":\"TOP\"},\"type\":\"ConnectorPlacement.EquallySpacedRectSide\",\"uuid\":\"ab9f1076-a7cc-4a5f-a71c-70d0f5e5f642\"}]},\"type\":\"ConnectorPlacement.EquallySpacedConnector\",\"uuid\":\"928155dc-f631-4629-bc1b-5a14a53f9ea7\"}],\"packageUris\":[\"http://schema.mathworks.com/mf0/Connector/R2020b\"],\"version\":\"1.0\"}"
  Front Right Hip : Subsystem
      settings: PortSchema="{\"entries\":[{\"content\":{\"sides\":[{\"content\":{\"connectorIds\":[\"LConn1\",\"LConn2\"]},\"type\":\"ConnectorPlacement.EquallySpacedRectSide\",\"uuid\":\"13a04993-3104-4ff0-9790-56bc88fd7271\"},{\"content\":{\"connectorIds\":[\"RConn1\"],\"side\":\"RIGHT\"},\"type\":\"ConnectorPlacement.EquallySpacedRectSide\",\"uuid\":\"d3121ca2-0bb7-489c-ba63-99aa3bb6178a\"},{\"content\":{\"connectorIds\":[\"LConn3\",\"LConn4\"],\"side\":\"TOP\"},\"type\":\"ConnectorPlacement.EquallySpacedRectSide\",\"uuid\":\"ab9f1076-a7cc-4a5f-a71c-70d0f5e5f642\"}]},\"type\":\"ConnectorPlacement.EquallySpacedConnector\",\"uuid\":\"928155dc-f631-4629-bc1b-5a14a53f9ea7\"}],\"packageUris\":[\"http://schema.mathworks.com/mf0/Connector/R2020b\"],\"version\":\"1.0\"}"
  Mux1 : Mux  Inputs=3
  Mux2 : Mux  Inputs=3
  PS-Simulink Converter{,1..5} (6 alike) : nesl_utility/PS-Simulink Converter  PhysicalDomain=network_engine_domain  SubClassName=ps_output  LeftPortType=input  RightPortType=output  PseudoPeriodic=off  Frequencies=[]  VectorFormat=inherit  Unit=inherit  AffineConversion=off
  Simulink-PS Converter : nesl_utility/Simulink-PS Converter  PhysicalDomain=network_engine_domain  SubClassName=ps_input  LeftPortType=input  RightPortType=output  PseudoPeriodic=off  Frequencies=[]  NoiseDistribution=none  NoiseParameters=[]  Unit=1  AffineConversion=off  FilteringAndDerivatives=provide  SimscapeFilterOrder=1  InputFilterTimeConstant=0.001  UdotUserProvided=0
  Simulink-PS Converter1 : nesl_utility/Simulink-PS Converter  PhysicalDomain=network_engine_domain  SubClassName=ps_input  LeftPortType=input  RightPortType=output  PseudoPeriodic=off  Frequencies=[]  NoiseDistribution=none  NoiseParameters=[]  Unit=1  AffineConversion=off  FilteringAndDerivatives=provide  SimscapeFilterOrder=1  InputFilterTimeConstant=0.001  UdotUserProvided=0
  Simulink-PS Converter2 : nesl_utility/Simulink-PS Converter  PhysicalDomain=network_engine_domain  SubClassName=ps_input  LeftPortType=input  RightPortType=output  PseudoPeriodic=off  Frequencies=[]  NoiseDistribution=none  NoiseParameters=[]  Unit=1  AffineConversion=off  FilteringAndDerivatives=provide  SimscapeFilterOrder=1  InputFilterTimeConstant=0.001  UdotUserProvided=0
  B : PMIOPort  Side=Left
  G : PMIOPort  Port=2  Side=Right
  FR_Foot_Frame : PMIOPort  Port=3  Side=Right
  q_FR : Outport
  dq_FR : Outport  Port=2
  wires:
  T_FR/1 -> Demux/1
  Demux/2 -> Simulink-PS Converter1/1
  Demux/1 -> Simulink-PS Converter/1
  Demux/3 -> Simulink-PS Converter2/1
  PS-Simulink Converter5/1 -> Mux2/3
  PS-Simulink Converter3/1 -> Mux2/1
  PS-Simulink Converter1/1 -> Mux1/2
  PS-Simulink Converter4/1 -> Mux2/2
  PS-Simulink Converter2/1 -> Mux1/3
  PS-Simulink Converter/1 -> Mux1/1
  Mux1/1 -> q_FR/1
  Mux2/1 -> dq_FR/1
  connections:
  Front Right Calf and Foot/LConn1 -- Front Right Thigh/RConn1
  Front Right Calf and Foot/RConn1 -- G/RConn1
  Front Right Hip/RConn1 -- Front Right Thigh/LConn1
  Front Right Hip/LConn1 -- B/RConn1
  Simulink-PS Converter/RConn1 -- Front Right Hip/LConn2
  Simulink-PS Converter1/RConn1 -- Front Right Thigh/LConn2
  Simulink-PS Converter2/RConn1 -- Front Right Calf and Foot/LConn2
  Front Right Calf and Foot/LConn4 -- PS-Simulink Converter5/LConn1
  Front Right Thigh/LConn4 -- PS-Simulink Converter4/LConn1
  Front Right Hip/LConn4 -- PS-Simulink Converter3/LConn1
  Front Right Calf and Foot/LConn3 -- PS-Simulink Converter2/LConn1
  Front Right Thigh/LConn3 -- PS-Simulink Converter1/LConn1
  Front Right Hip/LConn3 -- PS-Simulink Converter/LConn1
  FR_Foot_Frame/RConn1 -- Front Right Calf and Foot/RConn2

== system FinalProjectSimulinkModel_OBSTACLE/IMU ==
  imu_joint : sm_lib/Joints/Weld Joint  JointMode=Normal  SenseConstraintForce=off  SenseConstraintForceX=off  SenseConstraintForceY=off  SenseConstraintForceZ=off  SenseConstraintTorque=off  SenseConstraintTorqueX=off  SenseConstraintTorqueY=off  SenseConstraintTorqueZ=off  SenseTotalForce=off  SenseTotalForceX=off  SenseTotalForceY=off  SenseTotalForceZ=off  SenseTotalTorque=off  SenseTotalTorqueX=off  SenseTotalTorqueY=off  SenseTotalTorqueZ=off  CompositeWrenchDir=FollowerOnBase  CompositeWrenchFrame=BaseFrame
  imu_link : Subsystem
  B : PMIOPort  Side=Left
  connections:
  imu_joint/RConn1 -- imu_link/LConn1
  imu_joint/LConn1 -- B/RConn1

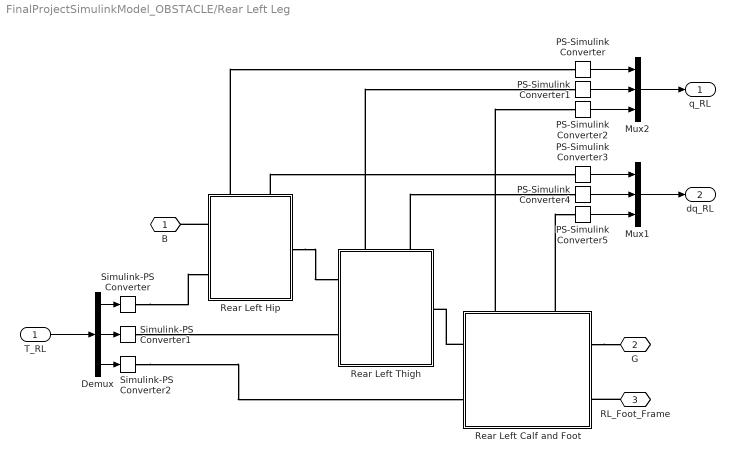
== system FinalProjectSimulinkModel_OBSTACLE/Rear Left Leg ==
  T_RL : Inport
  Demux : Demux  Outputs=3
  Mux1 : Mux  Inputs=3
  Mux2 : Mux  Inputs=3
  PS-Simulink Converter{,1..5} (6 alike) : nesl_utility/PS-Simulink Converter  PhysicalDomain=network_engine_domain  SubClassName=ps_output  LeftPortType=input  RightPortType=output  PseudoPeriodic=off  Frequencies=[]  VectorFormat=inherit  Unit=inherit  AffineConversion=off
  Rear Left Calf and Foot : Subsystem
      settings: PortSchema="{\"entries\":[{\"content\":{\"sides\":[{\"content\":{\"connectorIds\":[\"LConn1\",\"LConn2\"]},\"type\":\"ConnectorPlacement.EquallySpacedRectSide\",\"uuid\":\"13a04993-3104-4ff0-9790-56bc88fd7271\"},{\"content\":{\"connectorIds\":[\"RConn1\",\"RConn2\"],\"side\":\"RIGHT\"},\"type\":\"ConnectorPlacement.EquallySpacedRectSide\",\"uuid\":\"d3121ca2-0bb7-489c-ba63-99aa3bb6178a\"},{\"content\":{\"connectorIds\":[\"LConn3\",\"LConn4\"],\"side\":\"TOP\"},\"type\":\"ConnectorPlacement.EquallySpacedRectSide\",\"uuid\":\"ab9f1076-a7cc-4a5f-a71c-70d0f5e5f642\"}]},\"type\":\"ConnectorPlacement.EquallySpacedConnector\",\"uuid\":\"928155dc-f631-4629-bc1b-5a14a53f9ea7\"}],\"packageUris\":[\"http://schema.mathworks.com/mf0/Connector/R2020b\"],\"version\":\"1.0\"}"
  Rear Left Hip : Subsystem
      settings: PortSchema="{\"entries\":[{\"content\":{\"sides\":[{\"content\":{\"connectorIds\":[\"LConn1\",\"LConn2\"]},\"type\":\"ConnectorPlacement.EquallySpacedRectSide\",\"uuid\":\"13a04993-3104-4ff0-9790-56bc88fd7271\"},{\"content\":{\"connectorIds\":[\"RConn1\"],\"side\":\"RIGHT\"},\"type\":\"ConnectorPlacement.EquallySpacedRectSide\",\"uuid\":\"d3121ca2-0bb7-489c-ba63-99aa3bb6178a\"},{\"content\":{\"connectorIds\":[\"LConn3\",\"LConn4\"],\"side\":\"TOP\"},\"type\":\"ConnectorPlacement.EquallySpacedRectSide\",\"uuid\":\"ab9f1076-a7cc-4a5f-a71c-70d0f5e5f642\"}]},\"type\":\"ConnectorPlacement.EquallySpacedConnector\",\"uuid\":\"928155dc-f631-4629-bc1b-5a14a53f9ea7\"}],\"packageUris\":[\"http://schema.mathworks.com/mf0/Connector/R2020b\"],\"version\":\"1.0\"}"
  Rear Left Thigh : Subsystem
      settings: PortSchema="{\"entries\":[{\"content\":{\"sides\":[{\"content\":{\"connectorIds\":[\"LConn1\",\"LConn2\"]},\"type\":\"ConnectorPlacement.EquallySpacedRectSide\",\"uuid\":\"13a04993-3104-4ff0-9790-56bc88fd7271\"},{\"content\":{\"connectorIds\":[\"RConn1\"],\"side\":\"RIGHT\"},\"type\":\"ConnectorPlacement.EquallySpacedRectSide\",\"uuid\":\"d3121ca2-0bb7-489c-ba63-99aa3bb6178a\"},{\"content\":{\"connectorIds\":[\"LConn3\",\"LConn4\"],\"side\":\"TOP\"},\"type\":\"ConnectorPlacement.EquallySpacedRectSide\",\"uuid\":\"ab9f1076-a7cc-4a5f-a71c-70d0f5e5f642\"}]},\"type\":\"ConnectorPlacement.EquallySpacedConnector\",\"uuid\":\"928155dc-f631-4629-bc1b-5a14a53f9ea7\"}],\"packageUris\":[\"http://schema.mathworks.com/mf0/Connector/R2020b\"],\"version\":\"1.0\"}"
  Simulink-PS Converter : nesl_utility/Simulink-PS Converter  PhysicalDomain=network_engine_domain  SubClassName=ps_input  LeftPortType=input  RightPortType=output  PseudoPeriodic=off  Frequencies=[]  NoiseDistribution=none  NoiseParameters=[]  Unit=1  AffineConversion=off  FilteringAndDerivatives=provide  SimscapeFilterOrder=1  InputFilterTimeConstant=0.001  UdotUserProvided=0
  Simulink-PS Converter1 : nesl_utility/Simulink-PS Converter  PhysicalDomain=network_engine_domain  SubClassName=ps_input  LeftPortType=input  RightPortType=output  PseudoPeriodic=off  Frequencies=[]  NoiseDistribution=none  NoiseParameters=[]  Unit=1  AffineConversion=off  FilteringAndDerivatives=provide  SimscapeFilterOrder=1  InputFilterTimeConstant=0.001  UdotUserProvided=0
  Simulink-PS Converter2 : nesl_utility/Simulink-PS Converter  PhysicalDomain=network_engine_domain  SubClassName=ps_input  LeftPortType=input  RightPortType=output  PseudoPeriodic=off  Frequencies=[]  NoiseDistribution=none  NoiseParameters=[]  Unit=1  AffineConversion=off  FilteringAndDerivatives=provide  SimscapeFilterOrder=1  InputFilterTimeConstant=0.001  UdotUserProvided=0
  B : PMIOPort  Side=Left
  G : PMIOPort  Port=2  Side=Right
  RL_Foot_Frame : PMIOPort  Port=3  Side=Right
  q_RL : Outport
  dq_RL : Outport  Port=2
  wires:
  T_RL/1 -> Demux/1
  Demux/2 -> Simulink-PS Converter1/1
  Demux/1 -> Simulink-PS Converter/1
  Demux/3 -> Simulink-PS Converter2/1
  PS-Simulink Converter5/1 -> Mux1/3
  PS-Simulink Converter3/1 -> Mux1/1
  PS-Simulink Converter1/1 -> Mux2/2
  PS-Simulink Converter4/1 -> Mux1/2
  PS-Simulink Converter2/1 -> Mux2/3
  PS-Simulink Converter/1 -> Mux2/1
  Mux1/1 -> dq_RL/1
  Mux2/1 -> q_RL/1
  connections:
  Rear Left Hip/LConn1 -- B/RConn1
  Rear Left Calf and Foot/LConn1 -- Rear Left Thigh/RConn1
  Rear Left Calf and Foot/RConn1 -- G/RConn1
  Rear Left Hip/RConn1 -- Rear Left Thigh/LConn1
  Simulink-PS Converter/RConn1 -- Rear Left Hip/LConn2
  Simulink-PS Converter1/RConn1 -- Rear Left Thigh/LConn2
  Simulink-PS Converter2/RConn1 -- Rear Left Calf and Foot/LConn2
  Rear Left Hip/LConn3 -- PS-Simulink Converter/LConn1
  Rear Left Thigh/LConn3 -- PS-Simulink Converter1/LConn1
  Rear Left Calf and Foot/LConn3 -- PS-Simulink Converter2/LConn1
  Rear Left Hip/LConn4 -- PS-Simulink Converter3/LConn1
  Rear Left Thigh/LConn4 -- PS-Simulink Converter4/LConn1
  Rear Left Calf and Foot/LConn4 -- PS-Simulink Converter5/LConn1
  RL_Foot_Frame/RConn1 -- Rear Left Calf and Foot/RConn2
